simulink model "SNEO"  (R2020a)
settings: Solver=VariableStepAuto  StartTime=0.0  StopTime=30  RelTol=1e-3
libraries: dspfdesign x1, dspsigops x1
settings Model: Creator=diflo  LastModifiedBy=diflo

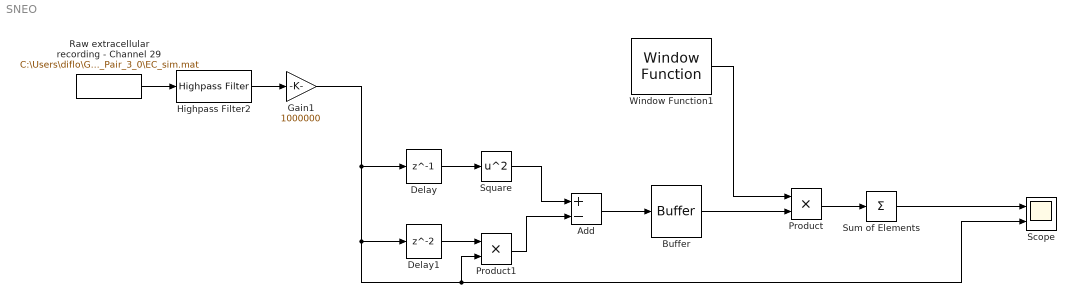
== system SNEO ==
  Add : Sum  Inputs=+-
  Buffer : Buffer  N=30  V=29  OutputFrames=off
  Delay : Delay  DelayLength=1  InitialCondition=0  SampleTime=1/30000
  Delay1 : Delay  InitialCondition=0  SampleTime=1/30000
  Gain1 : Gain  Gain=1000000
  Highpass Filter2 : dspfdesign/Highpass Filter  FilterType=IIR  DesignForMinimumOrder=off  FilterOrder=3  StopbandFrequency=1  PassbandFrequency=300  StopbandAttenuation=80  PassbandRipple=0.1  InheritSampleRate=off  SampleRate=30000  SimulateUsing=Interpreted execution  roundingMode=Floor  coeffsDataTypeStr=fixdt(1,16)
  Product : Product
  Product1 : Product
  Raw extracellular recording - Channel 29 : FromFile  FileName=C:\Users\diflo\Google Drive\IIT - Neuroengineering\MathWorks Project\Data\KampffLab\2014_11_25_Pair_3_0\EC_sim.mat  SampleTime=1/30000
  Scope : Scope  NumInputPorts=2
  Square : Math  Operator=square  SaturateOnIntegerOverflow=on
  Sum of Elements : Sum  Inputs=+
  Window Function1 : dspsigops/Window Function  winmode=Generate window  wintype=Hamming  sampmode=Discrete  samptime=1/30000  N=30  Rs=50  beta=10  winsamp=Symmetric  UserWindow=hamming  OptParams=off  UserParams={'symmetric'}  dataType=double  isSigned=on  wordLen=16  udDataType=sfix(16)  fracBitsMode=Best precision  numFracBits=15  roundingMode=Floor  overflowMode=off  numSidelobes=4  sidelobeLevel=-30
      settings: SourceProductBaseCode=DS
  wires:
  Raw extracellular recording - Channel 29/1 -> Highpass Filter2/1
  Gain1/1 -> Scope/2, Product1/2, Delay1/1, Delay/1
  Window Function1/1 -> Product/1
  Delay/1 -> Square/1
  Delay1/1 -> Product1/1
  Square/1 -> Add/1
  Product1/1 -> Add/2
  Add/1 -> Buffer/1
  Buffer/1 -> Product/2
  Product/1 -> Sum of Elements/1
  Highpass Filter2/1 -> Gain1/1
  Sum of Elements/1 -> Scope/1
